simulink model "Lab3_Model_Continuous"  (Simulink 8.7)
settings: Solver=VariableStepAuto  SolverMode=SingleTasking  StartTime=0.0  StopTime=10.0  RelTol=1e-3
values from neighbouring files (symbols this model uses):
  K1 = 0.66538    [Lab2.m]    (also in Lab3.m)
  K2 = 0.062    [Lab3.m]    (also in Lab3calculations.m)
  K3 = 4.78    [Lab3.m]    (also in Lab3calculations.m)
  Kp = 15    [Lab2.m]    (also in Lab3.m)
  Kp_c2 = 7    [Lab3.m]
  p = 10.5    [Lab2.m]    (also in Lab3.m)
  p_c2 = 2.5    [Lab3.m]
  tau = 0.030541    [Lab2.m]    (also in Lab3.m)
  z = 10    [Lab2.m]    (also in Lab3.m)
  z_c2 = 0.35    [Lab3.m]
settings Model: Creator=joe  LastModifiedBy=joe
settings DataIOCC: LimitDataPoints=off  SaveFormat=Dataset
settings DebuggingCC: UnderspecifiedInitializationDetection=Simplified  MergeDetectMultiDrivingBlocksExec=error  SFUnexpectedBacktrackingDiag=error  SFNoUnconditionalDefaultTransitionDiag=error
settings HardwareCC: ProdBitPerPointer=64  ProdLargestAtomicFloat=Float  ProdIntDivRoundTo=Zero  ProdEndianess=LittleEndian  ProdWordSize=64  ProdHWDeviceType=Intel->x86-64 (Windows64)
settings ModelReferenceCC: PropagateSignalLabelsOutOfModel=on
settings GRTTargetCC: TargetLangStandard=C99 (ISO)  GeneratePreprocessorConditionals=Use local settings
settings ConfigComp: CovMetricSettings=dwe  CovHtmlReporting=off  CovSaveCumulativeToWorkspaceVar=off  CovSaveSingleToWorkspaceVar=off  CovModelRefEnable=off  CovExternalEMLEnable=on

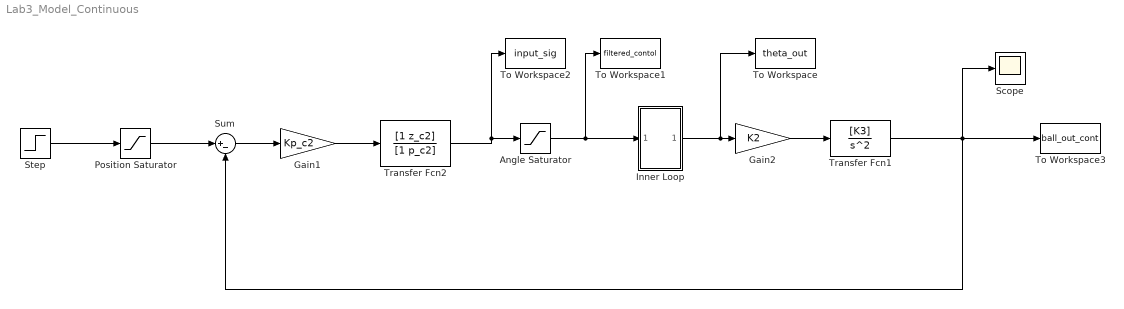
== system Lab3_Model_Continuous ==
  Angle Saturator : Saturate  UpperLimit=0.785  LowerLimit=-0.785
  Gain1 : Gain  Gain=Kp_c2
  Gain2 : Gain  Gain=K2
  Inner Loop : Subsystem
  Position Saturator : Saturate  UpperLimit=0.417  LowerLimit=0
  Scope : Scope
  Step : Step  Before=0.15  After=0.25  SampleTime=0
  Sum : Sum  Inputs=|+-
  To Workspace : ToWorkspace  VariableName=theta_out  SaveFormat=Timeseries  SampleTime=-1
  To Workspace1 : ToWorkspace  VariableName=filtered_contol  SaveFormat=Timeseries  SampleTime=-1
  To Workspace2 : ToWorkspace  VariableName=input_sig  SaveFormat=Timeseries  SampleTime=-1
  To Workspace3 : ToWorkspace  VariableName=ball_out_cont  SaveFormat=Timeseries  SampleTime=-1
  Transfer Fcn1 : TransferFcn  Numerator=[K3]  Denominator=[1 0 0]
  Transfer Fcn2 : TransferFcn  Numerator=[1 z_c2]  Denominator=[1 p_c2]
  wires:
  Transfer Fcn2/1 -> To Workspace2/1, Angle Saturator/1
  Angle Saturator/1 -> Inner Loop/1(In1), To Workspace1/1
  Gain1/1 -> Transfer Fcn2/1
  Sum/1 -> Gain1/1
  Position Saturator/1 -> Sum/1
  Step/1 -> Position Saturator/1
  Gain2/1 -> Transfer Fcn1/1
  Inner Loop/1(Out1) -> To Workspace/1, Gain2/1
  Transfer Fcn1/1 -> Sum/2, To Workspace3/1, Scope/1

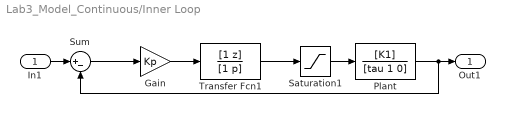
== system Lab3_Model_Continuous/Inner Loop ==
  In1 : Inport
  Gain : Gain  Gain=Kp
  Plant : TransferFcn  Numerator=[K1]  Denominator=[tau 1 0]
  Saturation1 : Saturate  UpperLimit=6  LowerLimit=-6
  Sum : Sum  Inputs=|+-
  Transfer Fcn1 : TransferFcn  Numerator=[1 z]  Denominator=[1 p]
  Out1 : Outport
  wires:
  In1/1 -> Sum/1
  Plant/1 -> Sum/2, Out1/1
  Gain/1 -> Transfer Fcn1/1
  Transfer Fcn1/1 -> Saturation1/1
  Sum/1 -> Gain/1
  Saturation1/1 -> Plant/1
